simulink subsystem "AnalyticFourBarLinkage"  (R2020b)
settings: Solver=VariableStepAuto  StartTime=0.0  StopTime=10.0  RelTol=1e-3
model mask{g=21, a=10.17, h=30.625, b=20.78, solutionSelector=1}
  mask prompts: g "g Distance between pivots"; a "a Length of crank arm"; h "h Length of coupler arm"; b "b Length of rocker arm"; solutionSelector "Solution number (1 or 2)"
settings Model: Creator=Edward  LastModifiedBy=Edward

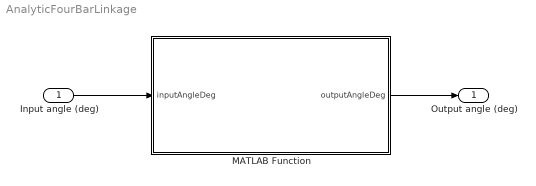
== system AnalyticFourBarLinkage ==
  Input angle (deg) : Inport
  MATLAB Function : MATLAB Function  TreatAsAtomicUnit=on
  Output angle (deg) : Outport
  wires:
  MATLAB Function/1(outputAngleDeg) -> Output angle (deg)/1
  Input angle (deg)/1 -> MATLAB Function/1(inputAngleDeg)

== matlab function AnalyticFourBarLinkage/MATLAB Function ==
  data: inputAngleDeg input; outputAngleDeg output; g parameter; b parameter; a parameter; h parameter; solutionSelector parameter
%g, b, a, h, solutionSelector are params from the sim (See "Edit Data"
%button in ribbon)
function outputAngleDeg = getOutputAngle(inputAngleDeg, g, b, a, h, solutionSelector)
assert(solutionSelector==1 || solutionSelector==2, "Solution selector must be 1 or 2");
outputAngleDegs = Mechanical.FourBarLinkage.getPossibleAnglesOfRightLinkageDegrees(g, b, a, h, inputAngleDeg);

outputAngleDeg = outputAngleDegs(solutionSelector);
end
